simulink model "neighobserver"  (R2021a)
settings: Solver=VariableStepAuto  StartTime=0.0  StopTime=20  RelTol=1e-3
values from neighbouring files (symbols this model uses):
  c = 1    [init_graph.m]
undefined symbols (not defined in the file or in its folder): A, B, B_dist, C1, C2, C3, C4, D, F1, F2, F3, F4, K, w1, w2
settings Model: Creator=umut  LastModifiedBy=umut

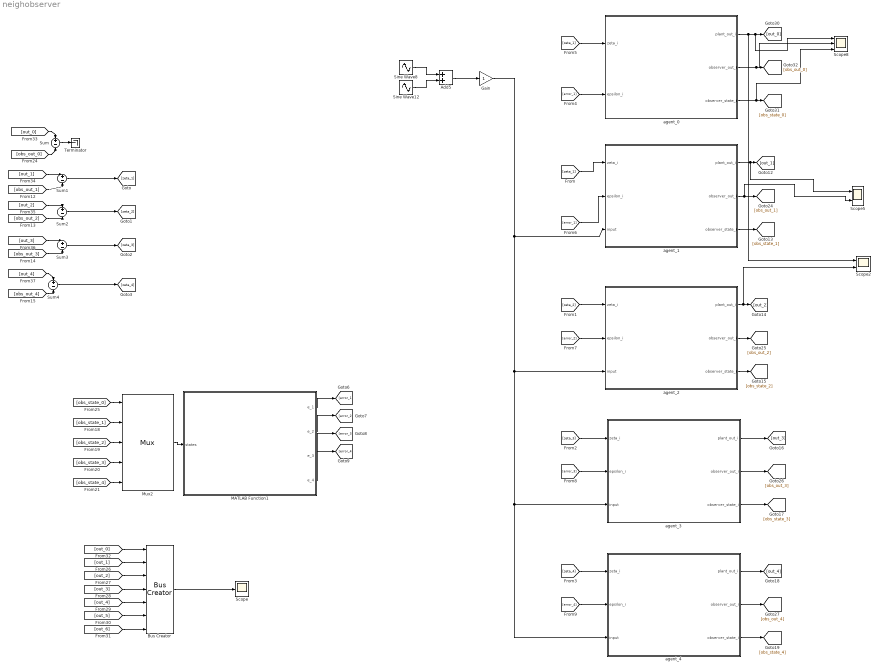
== system neighobserver ==
  Add5 : Sum
  Bus Creator : BusCreator  Inputs=7
  Gain : Gain
  MATLAB Function1 : MATLAB Function  TreatAsAtomicUnit=on
  Mux2 : Mux  Inputs=5
  Scope : Scope
  Scope2 : Scope  NumInputPorts=2
  Scope5 : Scope  NumInputPorts=2
  Scope8 : Scope  NumInputPorts=6
  Sine Wave12 : Sin  Amplitude=0.5  Frequency=w2  SampleTime=0
  Sine Wave8 : Sin  Amplitude=0.5  Frequency=w1  SampleTime=0
  Sum{,1..4} (5 alike) : Sum  Inputs=+|-
  Terminator : Terminator
  agent_0 : Subsystem
  agent_1 : Subsystem
  agent_2 : Subsystem
  agent_3 : Subsystem
  agent_4 : Subsystem
  wires:
  [obs_out_1] -> Sum1/2
  MATLAB Function1/2(e_2) -> [error_2]
  [out_3] -> Sum3/1
  [out_2] -> Sum2/1
  [out_1] -> Bus Creator/2
  [obs_out_2] -> Sum2/2
  Bus Creator/1 -> Scope/1
  [out_2] -> Bus Creator/3
  [obs_state_3] -> Mux2/4
  [obs_state_2] -> Mux2/3
  [out_4] -> Sum4/1
  [obs_state_1] -> Mux2/2
  [out_3] -> Bus Creator/4
  MATLAB Function1/4(e_4) -> [error_4]
  MATLAB Function1/3(e_3) -> [error_3]
  [out_4] -> Bus Creator/5
  Mux2/1 -> MATLAB Function1/1(states)
  MATLAB Function1/1(e_1) -> [error_1]
  [out_0] -> Sum/1
  [obs_out_0] -> Sum/2
  [out_1] -> Sum1/1
  [out_5] -> Bus Creator/6
  [out_0] -> Bus Creator/1
  [obs_state_0] -> Mux2/1
  [obs_out_4] -> Sum4/2
  [obs_out_3] -> Sum3/2
  [out_6] -> Bus Creator/7
  [obs_state_4] -> Mux2/5
  Sum4/1 -> [zeta_4]
  Sum3/1 -> [zeta_3]
  Sum2/1 -> [zeta_2]
  Sum1/1 -> [zeta_1]
  Sum/1 -> Terminator/1
  agent_4/3(observer_state_i) -> [obs_state_4]
  agent_4/1(plant_out_i) -> [out_4]
  [error_3] -> agent_3/2(epsilon_i)
  agent_2/1(plant_out_i) -> Scope2/2, [out_2]
  agent_0/3(observer_state_i) -> Scope8/6, [obs_state_0]
  agent_2/3(observer_state_i) -> [obs_state_2]
  agent_0/1(plant_out_i) -> Scope2/1, Scope8/1, [out_0]
  [zeta_1] -> agent_1/1(zeta_i)
  agent_3/1(plant_out_i) -> [out_3]
  [zeta_4] -> agent_4/1(zeta_i)
  [zeta_1] -> agent_0/1(zeta_i)
  [error_1] -> agent_1/2(epsilon_i)
  agent_4/2(observer_out_i) -> [obs_out_4]
  [zeta_3] -> agent_3/1(zeta_i)
  agent_1/3(observer_state_i) -> [obs_state_1]
  [error_2] -> agent_2/2(epsilon_i)
  [zeta_2] -> agent_2/1(zeta_i)
  [error_4] -> agent_4/2(epsilon_i)
  agent_3/3(observer_state_i) -> [obs_state_3]
  agent_0/2(observer_out_i) -> Scope8/3, [obs_out_0]
  agent_1/2(observer_out_i) -> Scope5/2, [obs_out_1]
  [error_1] -> agent_0/2(epsilon_i)
  agent_2/2(observer_out_i) -> [obs_out_2]
  agent_3/2(observer_out_i) -> [obs_out_3]
  Gain/1 -> agent_4/3(input), agent_3/3(input), agent_2/3(input), agent_1/3(input)
  agent_1/1(plant_out_i) -> Scope5/1, [out_1]
  Sine Wave8/1 -> Add5/1
  Add5/1 -> Gain/1
  Sine Wave12/1 -> Add5/2

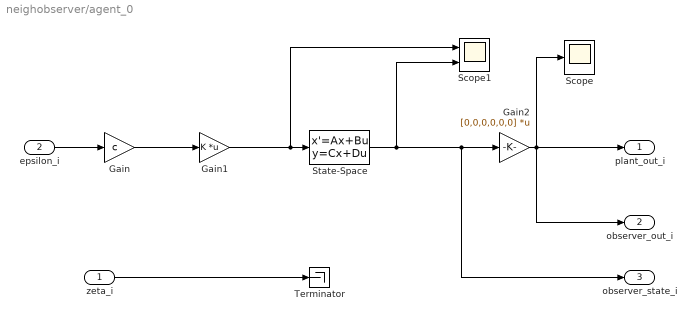
== system neighobserver/agent_0 ==
  zeta_i : Inport
  epsilon_i : Inport  Port=2
  Gain : Gain  Gain=c
  Gain1 : Gain  Gain=K  Multiplication=Matrix(K*u)
  Gain2 : Gain  Gain=[0,0,0,0,0,0]  Multiplication=Matrix(K*u)
  Scope : Scope
  Scope1 : Scope  NumInputPorts=2
  State-Space : StateSpace  A=A  B=B  C=zeros(6)  D=zeros(6,4)  InitialCondition=[0.1;0.2;0.3;0.4;0.5;0.6]
  Terminator : Terminator
  plant_out_i : Outport
  observer_out_i : Outport  Port=2
  observer_state_i : Outport  Port=3
  wires:
  epsilon_i/1 -> Gain/1
  zeta_i/1 -> Terminator/1
  State-Space/1 -> Scope1/2, Gain2/1, observer_state_i/1
  Gain/1 -> Gain1/1
  Gain2/1 -> Scope/1, plant_out_i/1, observer_out_i/1
  Gain1/1 -> Scope1/1, State-Space/1

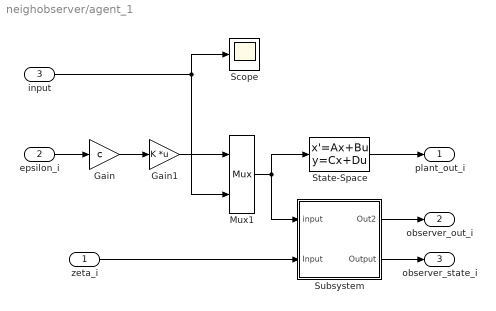
== system neighobserver/agent_1 ==
  zeta_i : Inport
  epsilon_i : Inport  Port=2
  input : Inport  Port=3
  Gain : Gain  Gain=c
  Gain1 : Gain  Gain=K  Multiplication=Matrix(K*u)
  Mux1 : Mux  Inputs=2
  Scope : Scope
  State-Space : StateSpace  A=A  B=[B B_dist]  C=C1  D=[D 0]  InitialCondition=[0.1;0.2;0.3;0.4;0.5;0.6]
  Subsystem : Subsystem
  plant_out_i : Outport
  observer_out_i : Outport  Port=2
  observer_state_i : Outport  Port=3
  wires:
  epsilon_i/1 -> Gain/1
  State-Space/1 -> plant_out_i/1
  Subsystem/1(Out2) -> observer_out_i/1
  Subsystem/2(Output) -> observer_state_i/1
  zeta_i/1 -> Subsystem/2(Input)
  Gain/1 -> Gain1/1
  Mux1/1 -> State-Space/1, Subsystem/1(input)
  Gain1/1 -> Mux1/1
  input/1 -> Scope/1, Mux1/2

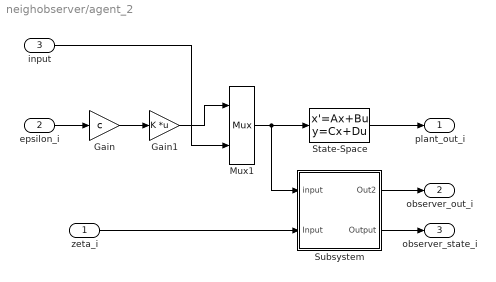
== system neighobserver/agent_2 ==
  zeta_i : Inport
  epsilon_i : Inport  Port=2
  input : Inport  Port=3
  Gain : Gain  Gain=c
  Gain1 : Gain  Gain=K  Multiplication=Matrix(K*u)
  Mux1 : Mux  Inputs=2
  State-Space : StateSpace  A=A  B=[B B_dist]  C=C2  D=[D 0]  InitialCondition=[0.6;0.5;0.4;0.3;0.2;0.1]
  Subsystem : Subsystem
  plant_out_i : Outport
  observer_out_i : Outport  Port=2
  observer_state_i : Outport  Port=3
  wires:
  epsilon_i/1 -> Gain/1
  State-Space/1 -> plant_out_i/1
  Subsystem/1(Out2) -> observer_out_i/1
  Subsystem/2(Output) -> observer_state_i/1
  zeta_i/1 -> Subsystem/2(Input)
  Gain/1 -> Gain1/1
  Mux1/1 -> Subsystem/1(input), State-Space/1
  Gain1/1 -> Mux1/1
  input/1 -> Mux1/2

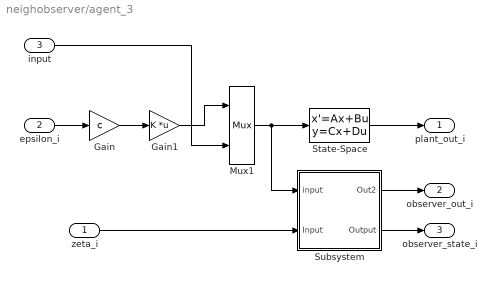
== system neighobserver/agent_3 ==
  zeta_i : Inport
  epsilon_i : Inport  Port=2
  input : Inport  Port=3
  Gain : Gain  Gain=c
  Gain1 : Gain  Gain=K  Multiplication=Matrix(K*u)
  Mux1 : Mux  Inputs=2
  State-Space : StateSpace  A=A  B=[B B_dist]  C=C3  D=[D 0]  InitialCondition=[0.6;0.3;0.1;0.4;0;0.8]
  Subsystem : Subsystem
  plant_out_i : Outport
  observer_out_i : Outport  Port=2
  observer_state_i : Outport  Port=3
  wires:
  epsilon_i/1 -> Gain/1
  State-Space/1 -> plant_out_i/1
  Subsystem/1(Out2) -> observer_out_i/1
  Subsystem/2(Output) -> observer_state_i/1
  zeta_i/1 -> Subsystem/2(Input)
  Gain/1 -> Gain1/1
  Mux1/1 -> Subsystem/1(input), State-Space/1
  Gain1/1 -> Mux1/1
  input/1 -> Mux1/2

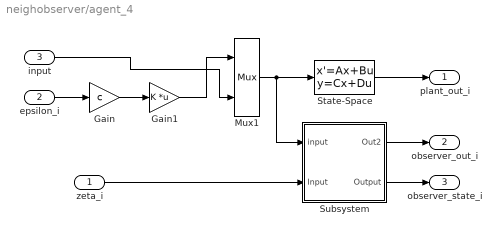
== system neighobserver/agent_4 ==
  zeta_i : Inport
  epsilon_i : Inport  Port=2
  input : Inport  Port=3
  Gain : Gain  Gain=c
  Gain1 : Gain  Gain=K  Multiplication=Matrix(K*u)
  Mux1 : Mux  Inputs=2
  State-Space : StateSpace  A=A  B=[B B_dist]  C=C4  D=[D 0]  InitialCondition=[0.3;0.1;0.7;0.2;0.8;0.4]
  Subsystem : Subsystem
  plant_out_i : Outport
  observer_out_i : Outport  Port=2
  observer_state_i : Outport  Port=3
  wires:
  epsilon_i/1 -> Gain/1
  State-Space/1 -> plant_out_i/1
  Subsystem/1(Out2) -> observer_out_i/1
  Subsystem/2(Output) -> observer_state_i/1
  zeta_i/1 -> Subsystem/2(Input)
  Gain/1 -> Gain1/1
  Mux1/1 -> Subsystem/1(input), State-Space/1
  Gain1/1 -> Mux1/1
  input/1 -> Mux1/2

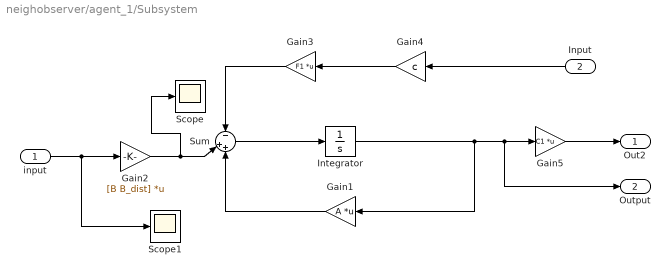
== system neighobserver/agent_1/Subsystem ==
  input : Inport
  Input : Inport  Port=2
  Gain1 : Gain  Gain=A  Multiplication=Matrix(K*u)
  Gain2 : Gain  Gain=[B B_dist]  Multiplication=Matrix(K*u)
  Gain3 : Gain  Gain=F1  Multiplication=Matrix(K*u)
  Gain4 : Gain  Gain=c
  Gain5 : Gain  Gain=C1  Multiplication=Matrix(K*u)
  Integrator : Integrator
  Scope : Scope
  Scope1 : Scope
  Sum : Sum  Inputs=-|++
  Out2 : Outport
  Output : Outport  Port=2
  wires:
  Gain3/1 -> Sum/1
  Gain2/1 -> Scope/1, Sum/2
  Gain1/1 -> Sum/3
  Sum/1 -> Integrator/1
  Gain5/1 -> Out2/1
  Input/1 -> Gain4/1
  Gain4/1 -> Gain3/1
  Integrator/1 -> Output/1, Gain5/1, Gain1/1
  input/1 -> Scope1/1, Gain2/1

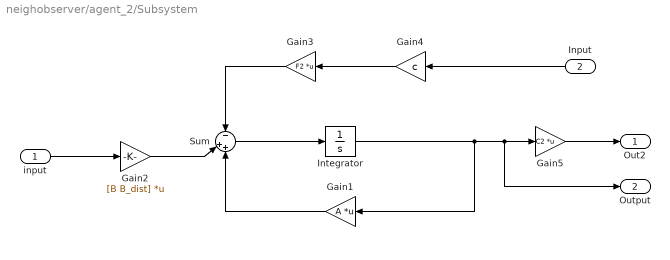
== system neighobserver/agent_2/Subsystem ==
  input : Inport
  Input : Inport  Port=2
  Gain1 : Gain  Gain=A  Multiplication=Matrix(K*u)
  Gain2 : Gain  Gain=[B B_dist]  Multiplication=Matrix(K*u)
  Gain3 : Gain  Gain=F2  Multiplication=Matrix(K*u)
  Gain4 : Gain  Gain=c
  Gain5 : Gain  Gain=C2  Multiplication=Matrix(K*u)
  Integrator : Integrator
  Sum : Sum  Inputs=-|++
  Out2 : Outport
  Output : Outport  Port=2
  wires:
  Gain3/1 -> Sum/1
  Gain2/1 -> Sum/2
  input/1 -> Gain2/1
  Gain1/1 -> Sum/3
  Sum/1 -> Integrator/1
  Gain5/1 -> Out2/1
  Input/1 -> Gain4/1
  Gain4/1 -> Gain3/1
  Integrator/1 -> Output/1, Gain5/1, Gain1/1

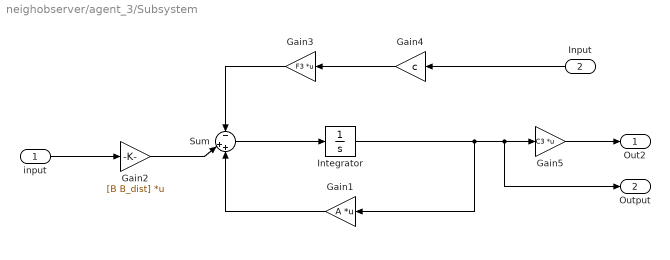
== system neighobserver/agent_3/Subsystem ==
  input : Inport
  Input : Inport  Port=2
  Gain1 : Gain  Gain=A  Multiplication=Matrix(K*u)
  Gain2 : Gain  Gain=[B B_dist]  Multiplication=Matrix(K*u)
  Gain3 : Gain  Gain=F3  Multiplication=Matrix(K*u)
  Gain4 : Gain  Gain=c
  Gain5 : Gain  Gain=C3  Multiplication=Matrix(K*u)
  Integrator : Integrator
  Sum : Sum  Inputs=-|++
  Out2 : Outport
  Output : Outport  Port=2
  wires:
  Gain3/1 -> Sum/1
  Gain2/1 -> Sum/2
  input/1 -> Gain2/1
  Gain1/1 -> Sum/3
  Sum/1 -> Integrator/1
  Gain5/1 -> Out2/1
  Input/1 -> Gain4/1
  Gain4/1 -> Gain3/1
  Integrator/1 -> Output/1, Gain5/1, Gain1/1

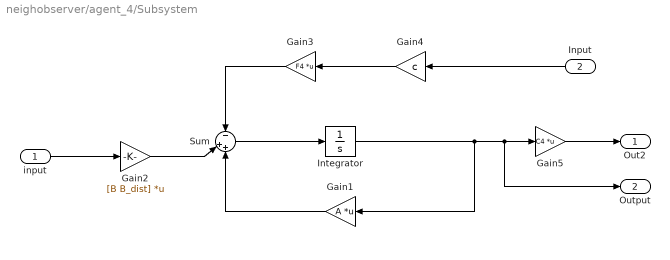
== system neighobserver/agent_4/Subsystem ==
  input : Inport
  Input : Inport  Port=2
  Gain1 : Gain  Gain=A  Multiplication=Matrix(K*u)
  Gain2 : Gain  Gain=[B B_dist]  Multiplication=Matrix(K*u)
  Gain3 : Gain  Gain=F4  Multiplication=Matrix(K*u)
  Gain4 : Gain  Gain=c
  Gain5 : Gain  Gain=C4  Multiplication=Matrix(K*u)
  Integrator : Integrator
  Sum : Sum  Inputs=-|++
  Out2 : Outport
  Output : Outport  Port=2
  wires:
  Gain3/1 -> Sum/1
  Gain2/1 -> Sum/2
  input/1 -> Gain2/1
  Gain1/1 -> Sum/3
  Sum/1 -> Integrator/1
  Gain5/1 -> Out2/1
  Input/1 -> Gain4/1
  Gain4/1 -> Gain3/1
  Integrator/1 -> Output/1, Gain5/1, Gain1/1

== matlab function neighobserver/MATLAB Function1 ==
  data: states input; e_1 output size=[4, 1]; e_2 output size=[4, 1]; e_3 output size=[4, 1]; e_4 output size=[4, 1]
function [e_1, e_2, e_3, e_4]  = calculate_neighborhood_error(states)
    adj = [ 0	0	0	0
            1   0   1   0
            1   0   0   1
            1   1   0   0]
    
    pinnings = [1; 0; 0; 0];

    A = adj;
    G = pinnings;
    
    size_agents = 4;
    size_states = 6;
    
    error = zeros(size_states, size_agents);
    
    
    for i = 1 : size_agents
        error_temp = [0;0;0;0;0;0];
        for j = 1 : size_agents
            error_temp = error_temp + A(i, j) * (states((j)*6+1 : 6*(j+1)) - states((i)*6+1 : 6*(i+1)));
        end
        error_temp = error_temp + pinnings(i) * (states(1 : 6) - states((i)*6+1 : 6*(i+1)));
        error(:,i) = error_temp;
    end
    
    e_1 = error(:,1);
    e_2 = error(:,2);
    e_3 = error(:,3);
    e_4 = error(:,4);

end
